simulink subsystem "SignalSnooping"  (R2026a)
settings: Solver=VariableStepAuto
libraries: uavmavlinklib x1
settings Model: Creator=The MathWorks, Inc.  LastModifiedBy=The MathWorks, Inc.

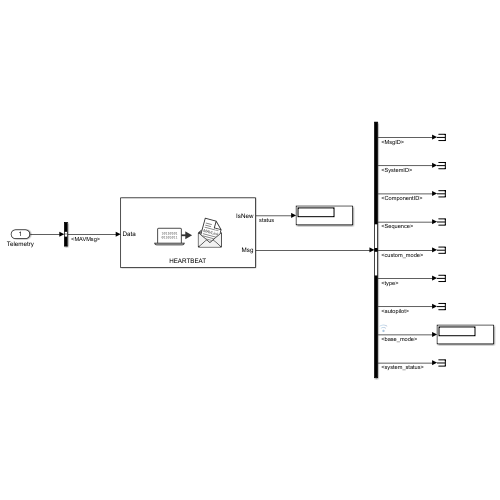
[thumbnail: Simulink's stored preview of the top-level diagram]
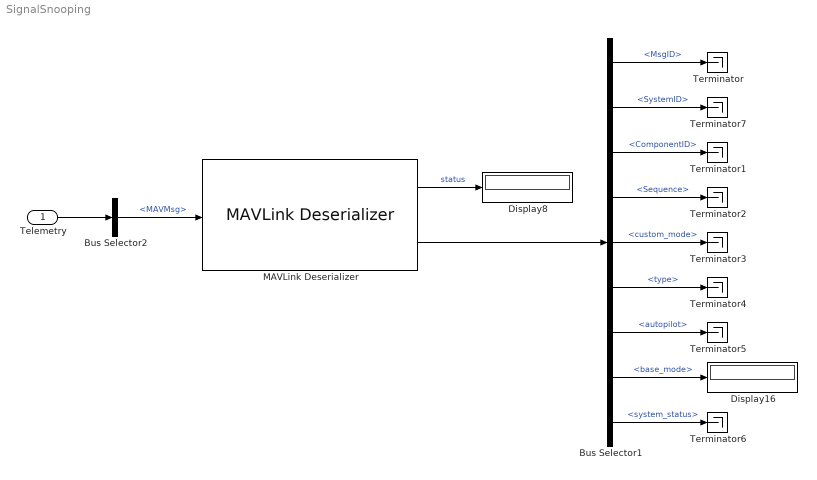
== system SignalSnooping ==
  Telemetry : Inport
  Bus Selector1 : BusSelector  OutputSignals=MsgID,SystemID,ComponentID,Sequence,Payload.custom_mode,Payload.type,Payload.autopilot,Payload.base_mode,Payload.system_status
  Bus Selector2 : BusSelector  OutputSignals=MAVMsg
  Display16 : Display
  Display8 : Display
  MAVLink Deserializer : uavmavlinklib/MAVLink Deserializer  dialectSource=Select from standard MAVLink dialects  dialect=common.xml  dialectCustom=common.xml  version=2  messageType=HEARTBEAT  inputDataLength=off  SystemIDFilter=off  systemID=1  ComponentIDFilter=off  componentID=1  queueMsg=off  queueMsgSize=50  dropNum=off
  Terminator{,1..7} (8 alike) : Terminator
  wires:
  Telemetry/1 -> Bus Selector2/1
  Bus Selector2/1 -> MAVLink Deserializer/1  "<MAVMsg>"
  MAVLink Deserializer/1 -> Display8/1  "status"
  MAVLink Deserializer/2 -> Bus Selector1/1
  Bus Selector1/8 -> Display16/1  "<base_mode>"
  Bus Selector1/1 -> Terminator/1  "<MsgID>"
  Bus Selector1/9 -> Terminator6/1  "<system_status>"
  Bus Selector1/7 -> Terminator5/1  "<autopilot>"
  Bus Selector1/6 -> Terminator4/1  "<type>"
  Bus Selector1/5 -> Terminator3/1  "<custom_mode>"
  Bus Selector1/4 -> Terminator2/1  "<Sequence>"
  Bus Selector1/3 -> Terminator1/1  "<ComponentID>"
  Bus Selector1/2 -> Terminator7/1  "<SystemID>"
